simulink model "ACC"  (Simulink 8.6)
settings: Solver=ode45  StartTime=0.0  StopTime=100  RelTol=1e-3
values from neighbouring files (symbols this model uses):
  a_w = 2    [Main.m]
  std = 2    [Main.m]
undefined symbols (not defined in the file or in its folder): sigbuilder_block
libraries: cstblocks x1
settings Model: Creator=cfloresp  LastModifiedBy=cfloresp
settings DebuggingCC: FcnCallInpInsideContextMsg=UseLocalSettings

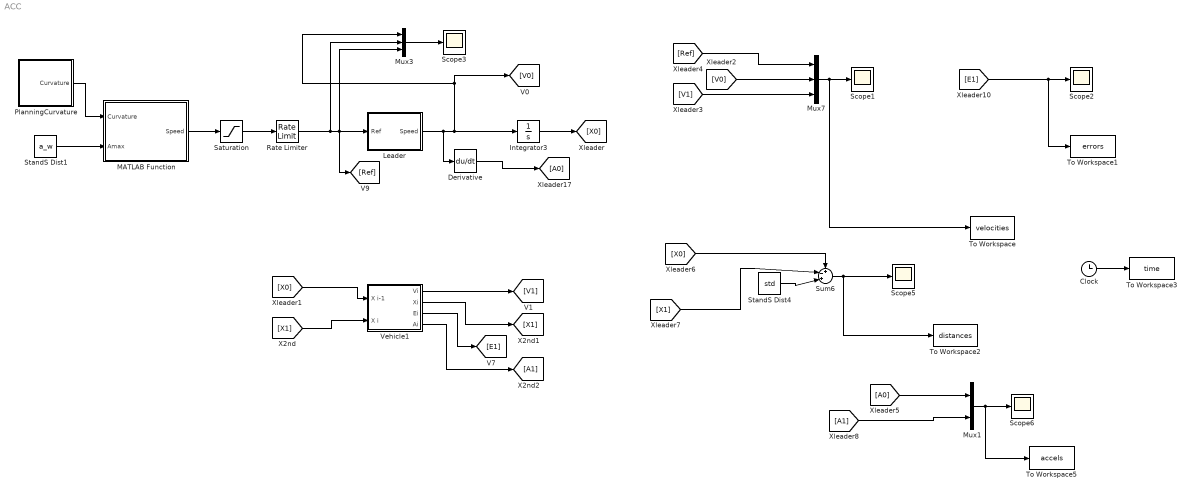
== system ACC ==
  Clock : Clock
  Derivative : Derivative
  Integrator3 : Integrator
  Leader : Subsystem
  MATLAB Function : MATLAB Function  TreatAsAtomicUnit=on
  Mux1 : Mux  Inputs=2
  Mux3 : Mux  Inputs=3
  Mux7 : Mux  Inputs=3
  PlanningCurvature : Subsystem
  Rate Limiter : RateLimiter  RisingSlewLimit=a_w  FallingSlewLimit=-a_w  SampleTimeMode=inherited
  Saturation : Saturate  UpperLimit=30  LowerLimit=0
  Scope{1..3,5..6} (5 alike) : Scope
  StandS Dist1 : Constant  Value=a_w
  StandS Dist4 : Constant  Value=std
  Sum6 : Sum  Inputs=+-+|
  To Workspace : ToWorkspace  VariableName=velocities  SampleTime=-1
  To Workspace1 : ToWorkspace  VariableName=errors  SampleTime=-1
  To Workspace2 : ToWorkspace  VariableName=distances  SampleTime=-1
  To Workspace3 : ToWorkspace  VariableName=time  SampleTime=-1
  To Workspace5 : ToWorkspace  VariableName=accels  SampleTime=-1
  Vehicle1 : Subsystem
  wires:
  Leader/1(Speed) -> Integrator3/1, [V0], Mux3/1, Derivative/1
  Integrator3/1 -> [X0]
  Sum6/1 -> Scope5/1, To Workspace2/1
  Rate Limiter/1 -> Mux3/2, Leader/1(Ref), Mux3/3, [Ref]
  [X0] -> Sum6/1
  [X1] -> Sum6/2
  [E1] -> Scope2/1, To Workspace1/1
  StandS Dist4/1 -> Sum6/3
  [X0] -> Vehicle1/1(X i-1)
  [X1] -> Vehicle1/2(X i)
  Vehicle1/1(Vi) -> [V1]
  Vehicle1/2(Xi) -> [X1]
  Vehicle1/3(Ei) -> [E1]
  Mux7/1 -> Scope1/1, To Workspace/1
  Mux3/1 -> Scope3/1
  Vehicle1/4(Ai) -> [A1]
  Clock/1 -> To Workspace3/1
  Derivative/1 -> [A0]
  [V1] -> Mux7/3
  [V0] -> Mux7/2
  [Ref] -> Mux7/1
  PlanningCurvature/1(Curvature) -> MATLAB Function/1(Curvature)
  StandS Dist1/1 -> MATLAB Function/2(Amax)
  MATLAB Function/1(Speed) -> Saturation/1
  Saturation/1 -> Rate Limiter/1
  Mux1/1 -> Scope6/1, To Workspace5/1
  [A0] -> Mux1/1
  [A1] -> Mux1/2

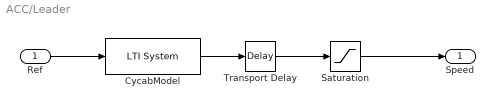
== system ACC/Leader ==
  Ref : Inport
  CycabModel : cstblocks/LTI System  sys=G_Veh  IC=[]
  Saturation : Saturate  UpperLimit=40  LowerLimit=0
  Transport Delay : TransportDelay  DelayTime=0
  Speed : Outport
  wires:
  Ref/1 -> CycabModel/1
  CycabModel/1 -> Transport Delay/1
  Saturation/1 -> Speed/1
  Transport Delay/1 -> Saturation/1

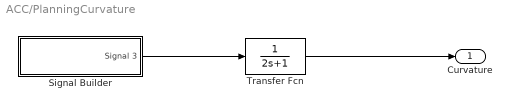
== system ACC/PlanningCurvature ==
  Signal Builder : Subsystem  Tag=STV Subsys  LoadFcn=sigbuilder_block('load');  StartFcn=sigbuilder_block('start');  StopFcn=sigbuilder_block('stop');  ClipboardFcn=sigbuilder_block('clipboard');  mask(Sigbuilder block){}
      mask help: Create and generate interchangeable groups of signals whose waveforms are piecewise linear.
      mask init:
      | if ~strcmp(get_param(bdroot(gcbh),'SimulationStatus'),'stopped') tuvar = sigbuilder_block('maskInit'); end
      settings: CopyFcn=sigbuilder_block('copy');  DeleteFcn=sigbuilder_block('delete');  ModelCloseFcn=sigbuilder_block('modelClose');  PreSaveFcn=sigbuilder_block('preSave');  PauseFcn=sigbuilder_block('pause')  ContinueFcn=sigbuilder_block('continue')  NameChangeFcn=sigbuilder_block('namechange');  OpenFcn=sigbuilder_block('open',[6 6 1428 741 ]);  CloseFcn=sigbuilder_block('close');
      mask Display: plot(0,0,100,100,[10,10,40,40,10],[80,20,20,80,80],[40,10],[50,50], [40,27,10],[65,72,56],[40,25,25,10],[28,28,43,43]);
  Transfer Fcn : TransferFcn  Denominator=[2 1]
  Curvature : Outport
  wires:
  Signal Builder/1(Signal 3) -> Transfer Fcn/1
  Transfer Fcn/1 -> Curvature/1

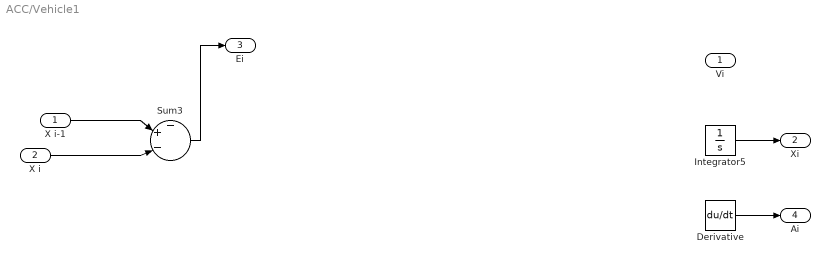
== system ACC/Vehicle1 ==
  X i-1 : Inport
  X i : Inport  Port=2
  Derivative : Derivative
  Integrator5 : Integrator
  Sum3 : Sum  Inputs=-+-|
  Vi : Outport
  Xi : Outport  Port=2
  Ei : Outport  Port=3
  Ai : Outport  Port=4
  wires:
  Sum3/1 -> Ei/1
  X i-1/1 -> Sum3/2
  Integrator5/1 -> Xi/1
  X i/1 -> Sum3/3
  Derivative/1 -> Ai/1

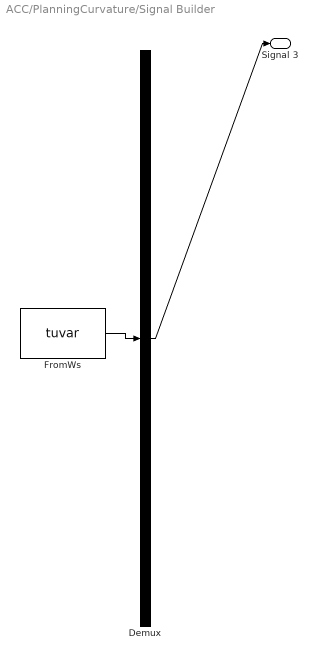
== system ACC/PlanningCurvature/Signal Builder ==
  Demux : Demux  Tag=STV Demux  Outputs=1
  FromWs : FromWorkspace  Tag=STV FromWs  VariableName=tuvar  SampleTime=0  SigBuilderData=DataTag0  VnvData=DataTag1
      SigBuilderData=|
      | common.afterFinalStr = 'Extrapolate'
      | common.sampleTime = 0
      | dataSet.timeRange = [0 100]
      | dataSet.name = 'Group 1'
      | sbobj.Groups.Name = 'Group 1'
      | sbobj.Groups.Signals.Name = 'Signal 3'
      | sbobj.Groups.Signals.XData = [0 0.53 0.53 9.36 14.83 19 25 30 33.67 55 60 65 70 85 95 100]
      | sbobj.Groups.Signals.YData = [-0.002 -0.002 0.001 0.316 0.316 0.142 -0.026 -0.026 0 0 -0.17 -0.172 0.078 0.076 0 0]
      | sbobj.Groups.TimeRange = [0 100]
  Signal 3 : Outport  Tag=STV Outport
  wires:
  FromWs/1 -> Demux/1
  Demux/1 -> Signal 3/1

== matlab function MATLAB Function ==
  data: Curvature input double; Speed output double; Amax input double
function Speed = MaxSpeed(Curvature, Amax)
%#codegen
